simulink model "PolePlacement_2019"  (R2022b)
settings: Solver=ode4  StartTime=0.0  StopTime=inf  FixedStep=0.002  RelTol=1e-3  EnableMultiTasking=on
PostLoadFcn:
  | qc_set_target_type(getConfigSet(bdroot, 'QUARC Default Target Configuration'));
values from neighbouring files (symbols this model uses):
  k = place(sysestc.A, sysestc.B, new_pole)    [PolePlacement.m]    (also in PolePlacement_Controller_script.m = place(A, B, new_pole); ppObs.m)
  Kr = 1/Kdc(1)    [PolePlacement.m]    (also in PolePlacement_Controller_script.m; ppObs.m)
  L = place(sysestc.A',sysestc.C', 10*new_pole)'    [PolePlacement.m]    (also in PolePlacement_Controller_script.m; ppObs.m)
  sysestc = d2c(sysest)    [PolePlacement.m]    (also in PolePlacement_Controller_script.m; ppObs.m)
undefined symbols (not defined in the file or in its folder): HIL, qc_get_step_size, sigbuilder_block
libraries: quarc_library x4
settings Model: SimulationMode=external  ExtModeTrigDuration=5000  Creator=CFulford  LastModifiedBy=AleFire
settings SolverCC: AlgebraicLoopSolver=TrustRegion  PositivePriorityOrder=on
settings DataIOCC: LimitDataPoints=on  SaveFormat=Array  SignalLoggingSaveFormat=ModelDataLogs  ReturnWorkspaceOutputs=off
settings OptimizationCC: ExpressionDepthLimit=2147483647  InitFltsAndDblsToZero=on  LifeSpan=inf
settings DebuggingCC: SaveWithParameterizedLinksMsg=none  UnderspecifiedInitializationDetection=Classic  MergeDetectMultiDrivingBlocksExec=none  SolverPrmCheckMsg=warning  MultiTaskDSMMsg=warning  MultiTaskCondExecSysMsg=none  FcnCallInpInsideContextMsg=warning  UnconnectedInputMsg=warning  UnconnectedOutputMsg=warning  UnconnectedLineMsg=warning  StateNameClashWarn=warning  SFUnexpectedBacktrackingDiag=warning  SFNoUnconditionalDefaultTransitionDiag=warning  SFExecutionAtInitializationDiag=none  SFMachineParentedDataDiag=warning  ArithmeticOperatorsInVariantConditions=warning
settings HardwareCC: ProdBitPerPointer=32  ProdBitPerSizeT=32  ProdBitPerPtrDiffT=32  ProdLargestAtomicFloat=None  ProdIntDivRoundTo=Undefined  ProdEndianess=Unspecified  ProdWordSize=32  ProdHWDeviceType=32-bit Generic
settings ModelReferenceCC: EnableRefExpFcnMdlSchedulingChecks=on  PropagateSignalLabelsOutOfModel=off
settings SFSimCC: SimUseLocalCustomCode=off  CustomCodeUndefinedFunction=UseInterfaceOnly
settings RTWCC: Description=QUARC Win64 Target  SystemTargetFile=quarc_win64.tlc  TemplateMakefile=quarc_default_tmf  RTWUseLocalCustomCode=off
settings CodeAppCC: StateflowObjectComments=on
settings STFCustomTargetCC: TargetPreCompLibLocation=C:\PROGRA~3\QUARC\lib\2019b\win64\release  ConcurrentExecutionCompliant=on  CombineOutputUpdateFcns=on  CPPClassGenCompliant=on  SystemTargetFile=quarc_win64.tlc
settings GRTTargetCC: TargetPreCompLibLocation=C:\PROGRA~3\QUARC\lib\2019b\win64\release  TargetLangStandard=C89/C90 (ANSI)  ParMdlRefBuildCompliant=off  CompOptLevelCompliant=off  MatFileLogging=off  UseToolchainInfoCompliant=off  ExtMode=on  ExtModeMexFile=quarc_comm
settings ConfigComp: CovMetricSettings=dw  CovSaveCumulativeToWorkspaceVar=on  CovSaveSingleToWorkspaceVar=on  CovExternalEMLEnable=off  CovSFcnEnable=off

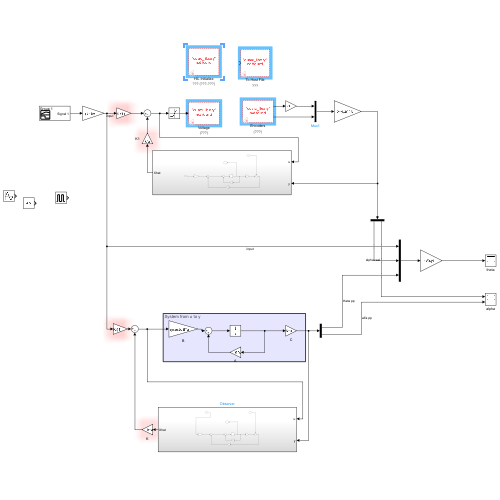
[thumbnail: Simulink's stored preview of the top-level diagram]
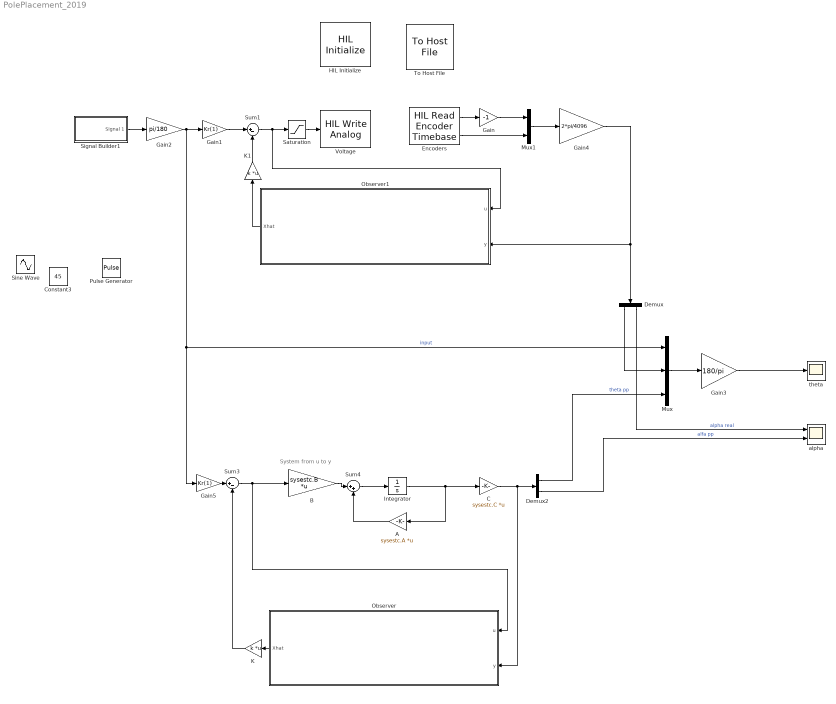
== system PolePlacement_2019 ==
  note: System from u to y
  A : Gain  Gain=sysestc.A  Multiplication=Matrix(K*u)
  B : Gain  Gain=sysestc.B  Multiplication=Matrix(K*u)
  C : Gain  Gain=sysestc.C  Multiplication=Matrix(K*u)
  Constant3 : Constant  Value=45
  Demux : Demux  Outputs=2
  Demux2 : Demux  Outputs=2
  Encoders : quarc_library/Data Acquisition/Generic/Timebases/HIL Read Encoder Timebase  object_name=HIL-1  clock=0  channels=[0:1]  samples_in_buffer=max(ceil(1/qc_get_step_size), 1)  active=on  vector_output=off  data_type_mode=Inherit via back propagation  data_type=double
  Gain : Gain  Gain=-1
  Gain1 : Gain  Gain=Kr(1)
  Gain2 : Gain  Gain=pi/180
  Gain3 : Gain  Gain=180/pi
  Gain4 : Gain  Gain=2*pi/4096
  Gain5 : Gain  Gain=Kr(1)
  HIL Initialize : quarc_library/Data Acquisition/Generic/Configuration/HIL Initialize  Priority=-99  object_name=HIL-1  board_type=q2_usb  board_number=0  board_options=d0=digital;d1=digital;led=auto;update_rate=normal;decimation=1  exclusive=off  active=off  hardware_clocks=[0]  clock_modes=[]  initial_clock_frequencies=[]  set_clock_params_at_start=off  set_clock_params_at_switch_in=off  set_clock_frequencies_at_start=off  set_clock_frequencies_at_switch_in=off  analog_input_channels=[0:1]  analog_input_configurations=[]  analog_input_maximums=10  analog_input_minimums=-10  set_analog_input_params_at_start=on  set_analog_input_params_at_switch_in=off  analog_output_channels=[0:1]  analog_output_maximums=10  analog_output_minimums=-10  initial_analog_outputs=[0]  final_analog_outputs=[0]  watchdog_analog_outputs=0  set_analog_output_params_at_start=on  set_analog_output_params_at_switch_in=off  set_analog_outputs_at_start=on  set_analog_outputs_at_switch_in=off  set_analog_outputs_at_terminate=on  set_analog_outputs_at_switch_out=off  set_analog_outputs_on_watchdog=off  digital_input_channels=[]  digital_output_channels=[]  digital_output_configuration=[]  initial_digital_outputs=[1]  final_digital_outputs=[1]  watchdog_digital_outputs=[1]  set_digital_output_params_at_start=off  set_digital_output_params_at_switch_in=off  set_digital_outputs_at_start=on  set_digital_outputs_at_switch_in=off  set_digital_outputs_at_terminate=on  set_digital_outputs_at_switch_out=off  set_digital_outputs_on_watchdog=off  encoder_channels=[0:1]  quadrature=[4]  encoder_filter_frequency=[]  initial_encoder_counts=[0]  set_encoder_params_at_start=on  set_encoder_params_at_switch_in=off  set_encoder_counts_at_start=on  set_encoder_counts_at_switch_in=off  pwm_channels=[]  pwm_modes=[0]  pwm_frequency=1/0.020  pwm_configuration=[]  pwm_alignment=[]  pwm_polarity=[]  pwm_leading_deadband=[]  pwm_trailing_deadband=[]  initial_pwm_outputs=[0]  final_pwm_outputs=[0]  watchdog_pwm_outputs=[0]  set_pwm_params_at_start=on  set_pwm_params_at_switch_in=off  set_pwm_outputs_at_start=on  set_pwm_outputs_at_switch_in=off  set_pwm_outputs_at_terminate=on  set_pwm_outputs_at_switch_out=off  set_pwm_outputs_on_watchdog=off  other_output_channels=[]  initial_other_outputs=[]  final_other_outputs=[]  watchdog_other_outputs=[]  set_other_outputs_at_start=off  set_other_outputs_at_switch_in=off  set_other_outputs_at_terminate=off  set_other_outputs_at_switch_out=off  set_other_outputs_on_watchdog=off
  Integrator : Integrator
  K : Gain  Gain=k  Multiplication=Matrix(K*u)
  K1 : Gain  Gain=k  Multiplication=Matrix(K*u)
  Mux : Mux  Inputs=3
  Mux1 : Mux  Inputs=2
  Observer : Subsystem
  Observer1 : Subsystem
  Pulse Generator : DiscretePulseGenerator  PulseType=Time based  Period=10  PulseWidth=5
  Saturation : Saturate  UpperLimit=5  LowerLimit=-5
  Signal Builder1 : Subsystem  Tag=STV Subsys  LoadFcn=sigbuilder_block('load');  StartFcn=sigbuilder_block('start');  StopFcn=sigbuilder_block('stop');  ClipboardFcn=sigbuilder_block('clipboard');  mask(Sigbuilder block){tuvar=[0:10]}
      mask help: Simulink:masks:SigbuilderBlock_MD
      mask init:
      | if ~strcmp(get_param(bdroot(gcbh),'SimulationStatus'),'stopped') tuvar = sigbuilder_block('maskInit'); end
      settings: CopyFcn=sigbuilder_block('copy');  DeleteFcn=sigbuilder_block('delete');  ModelCloseFcn=sigbuilder_block('modelClose');  PreSaveFcn=sigbuilder_block('preSave');  PauseFcn=sigbuilder_block('pause');  ContinueFcn=sigbuilder_block('continue');  NameChangeFcn=sigbuilder_block('namechange');  OpenFcn=sigbuilder_block('open',[437.6 199.2 550.4 400 ]);  CloseFcn=sigbuilder_block('close');
      mask Display: plot(0, 0, 100, 100,[2, 2, 32, 32, 2], [68, 8, 8, 68, 68],[32, 2], [38, 38], [32, 19, 2],[53, 60, 44], [32, 17, 17, 2],[16, 16, 31, 31]);txt = getActiveGroup(gcbh);text(2, 100, txt,'verticalAlignment', 'top');
  Sine Wave : Sin  Amplitude=45  Frequency=0.2*2*pi  SampleTime=0
  Sum1 : Sum  Inputs=|+-
  Sum3 : Sum  Inputs=|+-
  Sum4 : Sum  Inputs=|++
  To Host File : quarc_library/Sinks/To Host/To Host File  file_name=data_%{date}_%{time}.mat  variable_name=data_%{date}_%{time}  decimation=1  sample_time=0.002  file_format=MAT-file v.5  options=No header or footer  append=off  final_file_name=data_20-Mar-2023_17-30-44.mat  bitrate=2000000
  Voltage : quarc_library/Data Acquisition/Generic/Immediate I//O/HIL Write Analog  object_name=HIL-1  channels=0  sample_time=-1  active=off  vector_input=off
  alpha : Scope  NumInputPorts=2
  theta : Scope
  wires:
  Demux2/2 -> alpha/2  "alfa pp"
  K/1 -> Sum3/2
  Gain3/1 -> theta/1
  Demux2/1 -> Mux/3  "theta pp"
  Gain5/1 -> Sum3/1
  Observer/1(Xhat) -> K/1
  Mux/1 -> Gain3/1
  Sum3/1 -> Observer/1(u), B/1
  B/1 -> Sum4/1
  Gain2/1 -> Gain5/1, Mux/1, Gain1/1  "input"
  A/1 -> Sum4/2
  C/1 -> Demux2/1, Observer/2(y)
  Sum4/1 -> Integrator/1
  Integrator/1 -> A/1, C/1
  Observer1/1(Xhat) -> K1/1
  Gain1/1 -> Sum1/1
  Sum1/1 -> Saturation/1, Observer1/1(u)
  K1/1 -> Sum1/2
  Encoders/2 -> Mux1/2
  Encoders/1 -> Gain/1
  Mux1/1 -> Gain4/1
  Saturation/1 -> Voltage/1
  Gain4/1 -> Observer1/2(y), Demux/1
  Demux/1 -> Mux/2
  Demux/2 -> alpha/1  "alpha real"
  Gain/1 -> Mux1/1
  Signal Builder1/1(Signal 1) -> Gain2/1

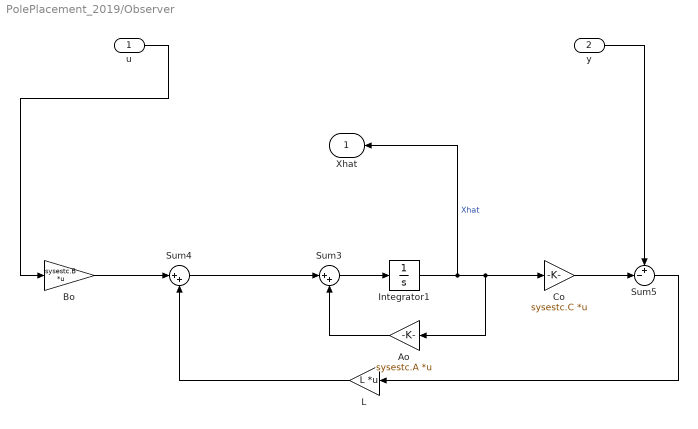
== system PolePlacement_2019/Observer ==
  u : Inport
  y : Inport  Port=2
  Ao : Gain  Gain=sysestc.A  Multiplication=Matrix(K*u)
  Bo : Gain  Gain=sysestc.B  Multiplication=Matrix(K*u)
  Co : Gain  Gain=sysestc.C  Multiplication=Matrix(K*u)
  Integrator1 : Integrator
  L : Gain  Gain=L  Multiplication=Matrix(K*u)
  Sum3 : Sum  Inputs=|++
  Sum4 : Sum  Inputs=|++
  Sum5 : Sum  Inputs=+-|
  Xhat : Outport
  wires:
  Sum5/1 -> L/1
  Sum4/1 -> Sum3/1
  u/1 -> Bo/1
  Sum3/1 -> Integrator1/1
  Integrator1/1 -> Xhat/1, Ao/1, Co/1  "Xhat"
  Ao/1 -> Sum3/2
  L/1 -> Sum4/2
  Co/1 -> Sum5/2
  Bo/1 -> Sum4/1
  y/1 -> Sum5/1

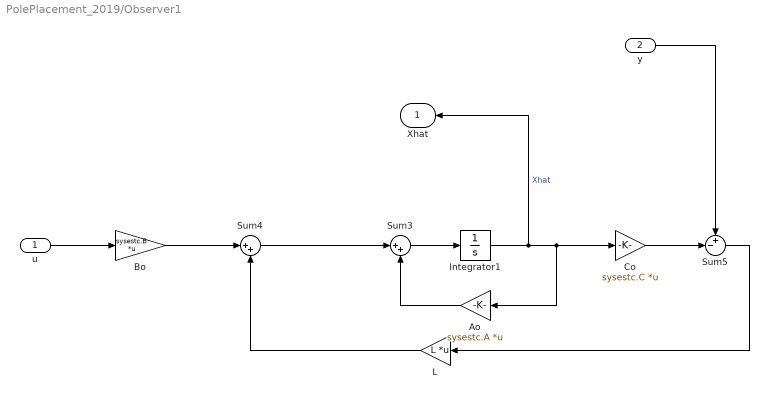
== system PolePlacement_2019/Observer1 ==
  u : Inport
  y : Inport  Port=2
  Ao : Gain  Gain=sysestc.A  Multiplication=Matrix(K*u)
  Bo : Gain  Gain=sysestc.B  Multiplication=Matrix(K*u)
  Co : Gain  Gain=sysestc.C  Multiplication=Matrix(K*u)
  Integrator1 : Integrator
  L : Gain  Gain=L  Multiplication=Matrix(K*u)
  Sum3 : Sum  Inputs=|++
  Sum4 : Sum  Inputs=|++
  Sum5 : Sum  Inputs=+-|
  Xhat : Outport
  wires:
  Sum5/1 -> L/1
  Sum4/1 -> Sum3/1
  u/1 -> Bo/1
  Sum3/1 -> Integrator1/1
  Integrator1/1 -> Xhat/1, Ao/1, Co/1  "Xhat"
  Ao/1 -> Sum3/2
  L/1 -> Sum4/2
  Co/1 -> Sum5/2
  Bo/1 -> Sum4/1
  y/1 -> Sum5/1

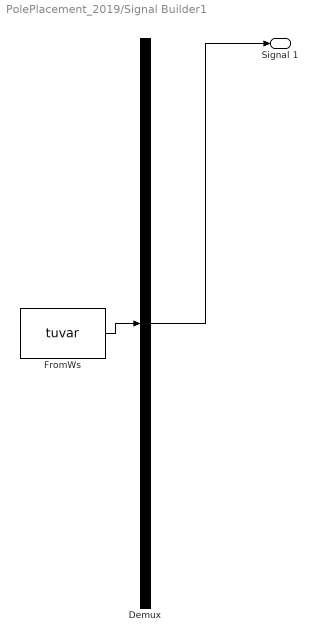
== system PolePlacement_2019/Signal Builder1 ==
  Demux : Demux  Tag=STV Demux  Outputs=1
      settings: DisplayOption=none
  FromWs : FromWorkspace  Tag=STV FromWs  VariableName=tuvar
      SigBuilderData=|
      | common.afterFinalStr = 'Extrapolate'
      | common.sampleTime = 0
      | dataSet.timeRange = [0 10]
      | dataSet.name = 'Group 1'
      | sbobj.Groups.Name = 'Group 1'
      | sbobj.Groups.Signals.Name = 'Signal 1'
      | sbobj.Groups.Signals.XData = [0 1 1 3 3 5 5 7 7 8.5 8.5 10]
      | sbobj.Groups.Signals.YData = [0.005 0.005 40 40 15 15 -30 -30 0 0 23 23]
  Signal 1 : Outport  Tag=STV Outport
  wires:
  Demux/1 -> Signal 1/1
  FromWs/1 -> Demux/1
